simulink model "cooked"  (R2024b)
settings: Solver=VariableStepAuto  StartTime=0.0  StopTime=50  RelTol=1e-3
model workspace (MAT data in the model file):
  w_1 = 5
settings Model: Creator=amlak  LastModifiedBy=amlak
settings DebuggingCC: AlgebraicLoopMsg=none

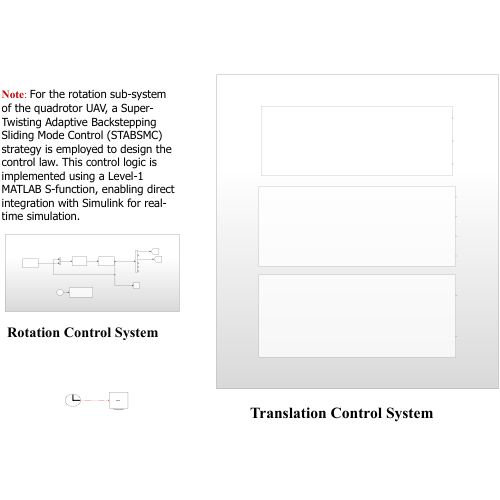
[thumbnail: Simulink's stored preview of the top-level diagram]
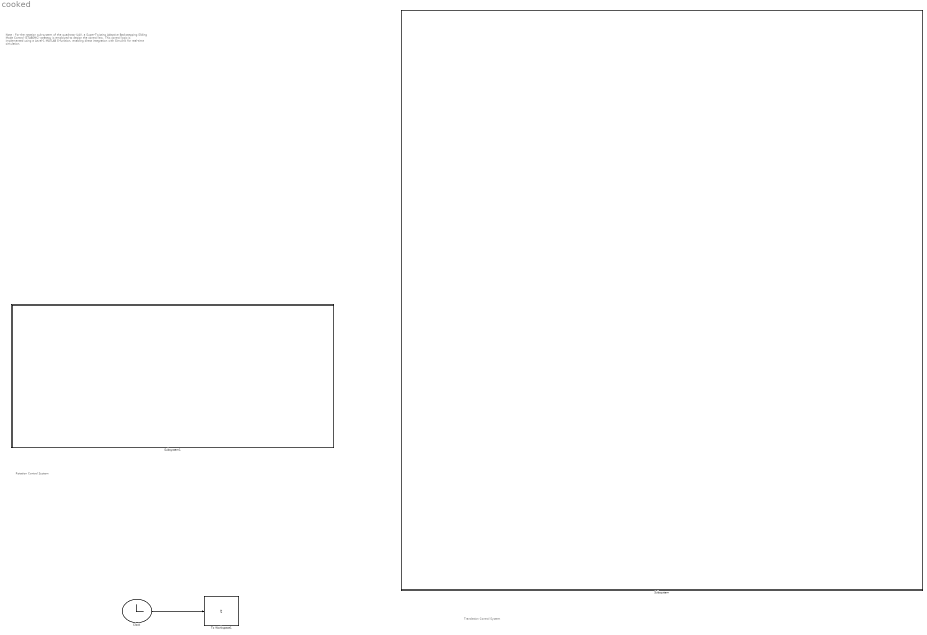
== system cooked ==
  note: Rotation Control System
  note: Note : For the rotation sub-system of the quadrotor UAV, a Super-Twisting Adaptive Backstepping Sliding Mode Control (STABSMC) strategy is employed to design the control law. This control logic is implemented using a Level-1 MATLAB S-function, enabling direct integration with Simulink for real-time simulation.
  note: Translation Control System
  Clock : Clock
      settings: Decimation=50
  Subsystem : Subsystem
  Subsystem1 : Subsystem
  To Workspace1 : ToWorkspace  VariableName=t  SampleTime=-1
      settings: Save2DSignal=2-D array (concatenate along first dimension)
  wires:
  Clock/1 -> To Workspace1/1

== system cooked/Subsystem ==
  Subsystem1 : Subsystem
  Subsystem2 : Subsystem
  Subsystem4 : Subsystem

== system cooked/Subsystem1 ==
  Clock1 : Clock
      settings: Decimation=50
  Demux : Demux  Outputs=6
  Mux1 : Mux  Inputs=2
  S-Function : S-Function  FunctionName=input_qpr  SFunctionDeploymentMode=off  EnableBusSupport=off
  S-Function1 : S-Function  FunctionName=control_qpr  SFunctionDeploymentMode=off  EnableBusSupport=off
  S-Function2 : S-Function  FunctionName=plant_pqr  SFunctionDeploymentMode=off  EnableBusSupport=off
  Scope1 : Scope
  To Workspace : ToWorkspace  VariableName=simout  SaveFormat=Timeseries  SampleTime=-1
  tag scope: x1=global, x3=global
  wires:
  S-Function/1 -> Mux1/2
  Mux1/1 -> S-Function1/1
  Clock1/1 -> To Workspace/1
  S-Function2/1 -> Mux1/1, Scope1/1, Demux/1
  S-Function1/1 -> S-Function2/1
  Demux/3 -> [x3]
  Demux/1 -> [x1]

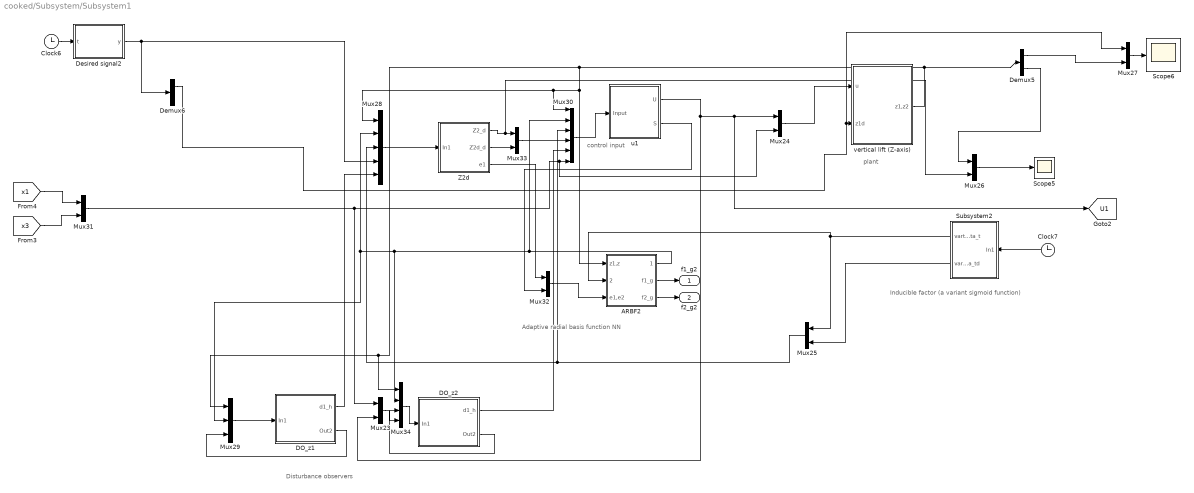
== system cooked/Subsystem/Subsystem1 ==
  note: control input
  note: Inducible factor (a variant sigmoid function)
  note: plant
  note: Disturbance observers
  note: Adaptive radial basis function NN
  ARBF2 : Subsystem
  Clock6 : Clock
      settings: Decimation=50
  Clock7 : Clock
      settings: Decimation=50
  DO_z1 : Subsystem
  DO_z2 : Subsystem
  Demux5 : Demux  Outputs=2
  Demux6 : Demux  Outputs=2
  Desired signal2 : MATLAB Function  TreatAsAtomicUnit=on
  Mux{23..27,31..33} (8 alike) : Mux  Inputs=2
  Mux28 : Mux  Inputs=5
  Mux29 : Mux  Inputs=3
  Mux30 : Mux  Inputs=6
  Mux34 : Mux
  Scope5 : Scope
  Scope6 : Scope
  Subsystem2 : Subsystem
  Z2d : Subsystem
  u1 : Subsystem
  vertical lift (Z-axis) : Subsystem
  f1_g2 : Outport
  f2_g2 : Outport  Port=2
  tag scope: U1=global
  wires:
  u1/1(U) -> Mux23/2, [U1], Mux24/1
  Z2d/3(e1) -> Mux32/1
  vertical lift (Z-axis)/1(z1,z2) -> Mux28/1, Mux30/1, ARBF2/1(z1,z), Mux34/1, Mux29/1, Demux5/1
  Mux26/1 -> Scope5/1
  Mux31/1 -> Mux24/2, Mux30/6, Mux23/1
  ARBF2/2(f1_g) -> f1_g2/1
  Mux24/1 -> vertical lift (Z-axis)/1(u)
  ARBF2/1(lambda) -> Mux30/2, Mux28/2, Mux29/2, Mux34/2
  ARBF2/3(f2_g) -> f2_g2/1
  DO_z2/1(d1_h) -> Mux30/5
  Subsystem2/1(vartheta_t) -> ARBF2/2(vartheta_t), Mux25/1
  Demux5/2 -> Mux26/1
  DO_z1/1(d1_h) -> Mux28/5
  Mux33/1 -> Mux30/4
  Mux32/1 -> ARBF2/3(e1,e2)
  Demux6/1 -> Mux27/1, vertical lift (Z-axis)/2(z1d)
  Mux30/1 -> u1/1(Input)
  Mux28/1 -> Z2d/1(In1)
  Clock7/1 -> Subsystem2/1(In1)
  Z2d/2(Z2d_d) -> Mux33/2
  [x1] -> Mux31/1
  Mux23/1 -> Mux34/4
  DO_z2/2(Out2) -> Mux34/3
  Desired signal2/1(y) -> Demux6/1, Mux28/4
  Mux34/1 -> DO_z2/1(In1)
  Subsystem2/2(vartheta_td) -> Mux25/2
  [x3] -> Mux31/2
  Mux27/1 -> Scope6/1
  Mux29/1 -> DO_z1/1(In1)
  DO_z1/2(Out2) -> Mux29/3
  Z2d/1(Z2_d) -> Mux26/2, Mux33/1
  u1/2(S) -> Mux32/2
  Clock6/1 -> Desired signal2/1(t)
  Demux5/1 -> Mux27/2
  Mux25/1 -> Mux28/3, Mux30/3

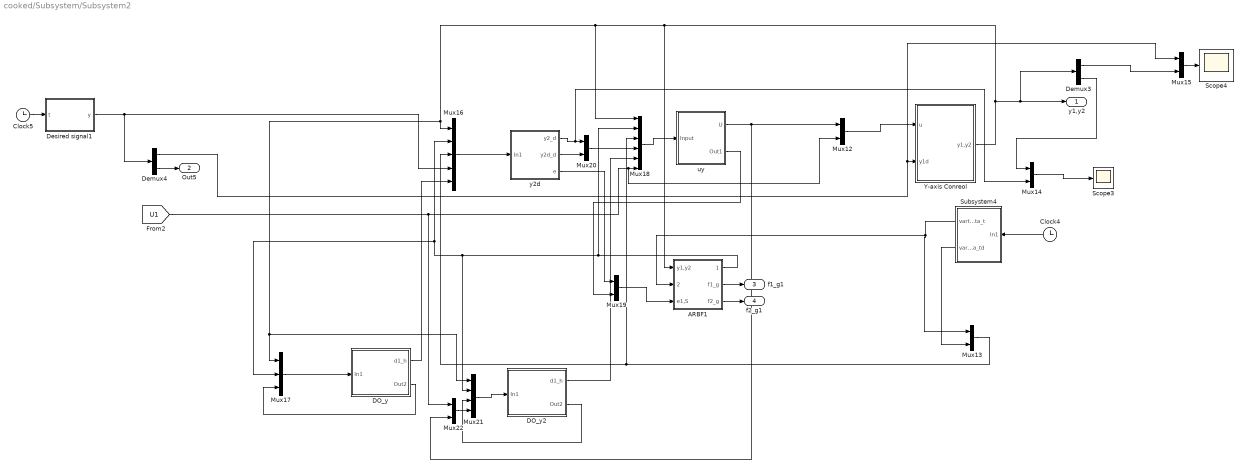
== system cooked/Subsystem/Subsystem2 ==
  ARBF1 : Subsystem
  Clock4 : Clock
      settings: Decimation=50
  Clock5 : Clock
      settings: Decimation=50
  DO_y : Subsystem
  DO_y2 : Subsystem
  Demux3 : Demux  Outputs=2
  Demux4 : Demux  Outputs=2
  Desired signal1 : MATLAB Function  TreatAsAtomicUnit=on
  Mux{12..15,19..20,22} (7 alike) : Mux  Inputs=2
  Mux16 : Mux  Inputs=5
  Mux17 : Mux  Inputs=3
  Mux18 : Mux  Inputs=6
  Mux21 : Mux
  Scope3 : Scope
  Scope4 : Scope
  Subsystem4 : Subsystem
  Y-axis Conreol : Subsystem
  uy : Subsystem
  y2d : Subsystem
  y1,y2 : Outport
  Out5 : Outport  Port=2
  f1_g1 : Outport  Port=3
  f2_g1 : Outport  Port=4
  wires:
  DO_y2/2(Out2) -> Mux21/3
  ARBF1/3(f2_g) -> f2_g1/1
  Mux19/1 -> ARBF1/3(e1,S)
  Clock5/1 -> Desired signal1/1(t)
  Subsystem4/1(vartheta_t) -> Mux13/1, ARBF1/2(vartheta_t)
  Mux16/1 -> y2d/1(In1)
  ARBF1/1(lambda) -> Mux18/2, Mux21/2, Mux17/2, Mux16/2
  Y-axis Conreol/1(y1,y2) -> y1,y2/1, Demux3/1, ARBF1/1(y1,y2), Mux18/1, Mux21/1, Mux17/1, Mux16/1
  Desired signal1/1(y) -> Demux4/1, Mux16/4
  Demux3/2 -> Mux14/1
  Demux4/2 -> Out5/1
  Mux21/1 -> DO_y2/1(In1)
  Mux18/1 -> uy/1(Input)
  [U1] -> Mux12/2, Mux18/6, Mux22/1
  Mux14/1 -> Scope3/1
  Mux17/1 -> DO_y/1(In1)
  y2d/2(y2d_d) -> Mux20/2
  Mux22/1 -> Mux21/4
  Mux13/1 -> Mux16/3, Mux18/3
  y2d/1(y2_d) -> Mux14/2, Mux20/1
  Demux4/1 -> Mux15/1, Y-axis Conreol/2(y1d)
  uy/1(U) -> Mux22/2, Mux12/1
  y2d/3(e) -> Mux19/1
  Clock4/1 -> Subsystem4/1(In1)
  Demux3/1 -> Mux15/2
  DO_y/1(d1_h) -> Mux16/5
  Subsystem4/2(vartheta_td) -> Mux13/2
  DO_y/2(Out2) -> Mux17/3
  Mux20/1 -> Mux18/4
  ARBF1/2(f1_g) -> f1_g1/1
  DO_y2/1(d1_h) -> Mux18/5
  uy/2(Out1) -> Mux19/2
  Mux15/1 -> Scope4/1
  Mux12/1 -> Y-axis Conreol/1(u)

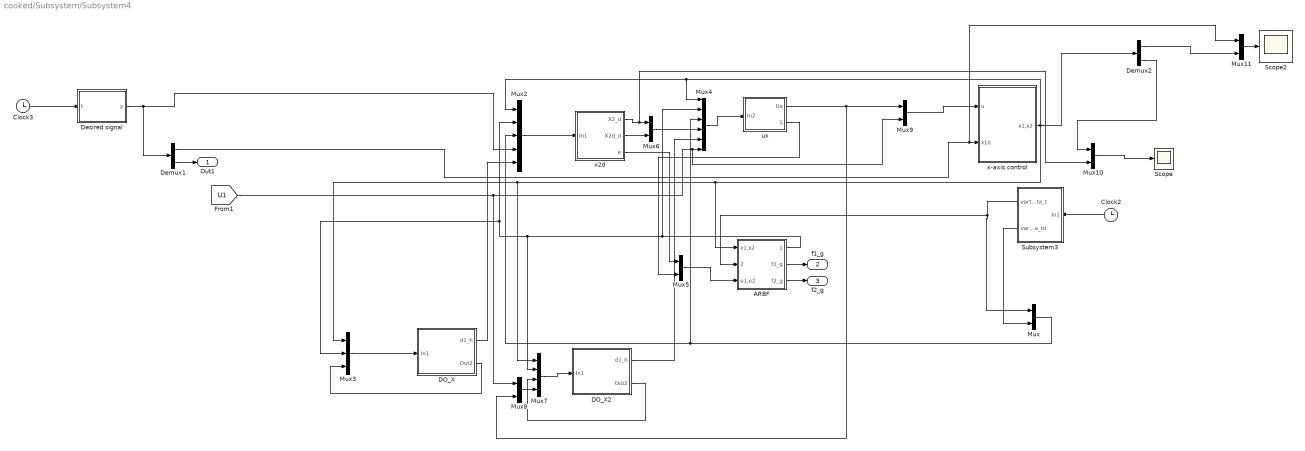
== system cooked/Subsystem/Subsystem4 ==
  ARBF : Subsystem
  Clock2 : Clock
      settings: Decimation=50
  Clock3 : Clock
      settings: Decimation=50
  DO_X : Subsystem
  DO_X2 : Subsystem
  Demux1 : Demux  Outputs=2
  Demux2 : Demux  Outputs=2
  Desired signal : MATLAB Function  TreatAsAtomicUnit=on
  Mux{,5..6,8..11} (7 alike) : Mux  Inputs=2
  Mux2 : Mux  Inputs=5
  Mux3 : Mux  Inputs=3
  Mux4 : Mux  Inputs=6
  Mux7 : Mux
  Scope : Scope
  Scope2 : Scope
  Subsystem3 : Subsystem
  ux : Subsystem
  x-axis control : Subsystem
  x2d : Subsystem
  Out1 : Outport
  f1_g : Outport  Port=2
  f2_g : Outport  Port=3
  wires:
  DO_X/2(Out2) -> Mux3/3
  Mux10/1 -> Scope/1
  ARBF/3(f2_g) -> f2_g/1
  ARBF/1(lambda) -> Mux4/2, Mux7/2, Mux3/2, Mux2/2
  Demux2/2 -> Mux10/1
  Mux3/1 -> DO_X/1(In1)
  Subsystem3/1(vartheta_t) -> Mux/1, ARBF/2(vartheta_t)
  Demux1/1 -> Mux11/1, x-axis control/2(x1d)
  Desired signal/1(y) -> Demux1/1, Mux2/4
  Demux1/2 -> Out1/1
  DO_X2/1(d1_h) -> Mux4/5
  x-axis control/1(x1,x2) -> Mux7/1, Mux3/1, ARBF/1(x1,x2), Demux2/1, Mux2/1, Mux4/1
  DO_X2/2(Out2) -> Mux7/3
  ux/2(S) -> Mux5/2
  [U1] -> Mux9/2, Mux4/6, Mux8/1
  Demux2/1 -> Mux11/2
  Mux5/1 -> ARBF/3(e1,e2)
  Mux9/1 -> x-axis control/1(u)
  Mux2/1 -> x2d/1(In1)
  Subsystem3/2(vartheta_td) -> Mux/2
  Clock3/1 -> Desired signal/1(t)
  DO_X/1(d1_h) -> Mux2/5
  x2d/1(X2_d) -> Mux10/2, Mux6/1
  Mux7/1 -> DO_X2/1(In1)
  x2d/2(X2d_d) -> Mux6/2
  ARBF/2(f1_g) -> f1_g/1
  Mux4/1 -> ux/1(In2)
  Mux6/1 -> Mux4/4
  ux/1(Ux) -> Mux9/1, Mux8/2
  Mux11/1 -> Scope2/1
  Mux8/1 -> Mux7/4
  Mux/1 -> Mux2/3, Mux4/3
  Clock2/1 -> Subsystem3/1(In1)
  x2d/3(e) -> Mux5/1

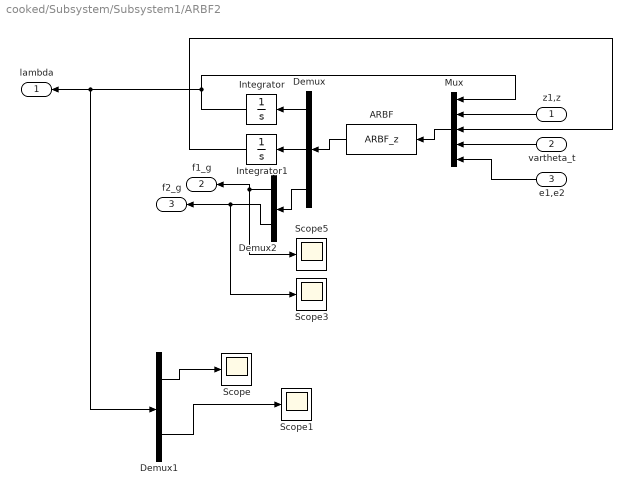
== system cooked/Subsystem/Subsystem1/ARBF2 ==
  z1,z : Inport
  vartheta_t : Inport  Port=2
  e1,e2 : Inport  Port=3
  ARBF : MATLABFcn  MATLABFcn=ARBF_z  OutputDimensions=42
  Demux : Demux  Outputs=[2 38 2]
  Demux1 : Demux  Outputs=2
  Demux2 : Demux  Outputs=2
  Integrator : Integrator
  Integrator1 : Integrator
  Mux : Mux  Inputs=5
  Scope{,1,3,5} (4 alike) : Scope
  lambda : Outport
  f1_g : Outport  Port=2
  f2_g : Outport  Port=3
  wires:
  ARBF/1 -> Demux/1
  Mux/1 -> ARBF/1
  Demux2/1 -> f1_g/1, Scope5/1
  Demux2/2 -> f2_g/1, Scope3/1
  Demux1/1 -> Scope/1
  Demux/1 -> Integrator/1
  Demux/3 -> Demux2/1
  z1,z/1 -> Mux/2
  e1,e2/1 -> Mux/5
  Integrator/1 -> lambda/1, Demux1/1, Mux/1
  Demux/2 -> Integrator1/1
  Demux1/2 -> Scope1/1
  Integrator1/1 -> Mux/3
  vartheta_t/1 -> Mux/4

== system cooked/Subsystem/Subsystem1/DO_z1 ==
  In1 : Inport
  DO1 : MATLABFcn  MATLABFcn=DO_z  OutputDimensions=2
  Demux : Demux  Outputs=2
  Integrator : Integrator
  Scope : Scope
  d1_h : Outport
  Out2 : Outport  Port=2
  wires:
  Demux/2 -> Integrator/1
  DO1/1 -> Demux/1
  In1/1 -> DO1/1
  Integrator/1 -> Out2/1
  Demux/1 -> Scope/1, d1_h/1

== system cooked/Subsystem/Subsystem1/DO_z2 ==
  In1 : Inport
  DO_x2 : MATLABFcn  MATLABFcn=DO_z2  OutputDimensions=2
  Demux : Demux  Outputs=2
  Integrator : Integrator
  d1_h : Outport
  Out2 : Outport  Port=2
  wires:
  Demux/1 -> d1_h/1
  Demux/2 -> Integrator/1
  DO_x2/1 -> Demux/1
  In1/1 -> DO_x2/1
  Integrator/1 -> Out2/1

== system cooked/Subsystem/Subsystem1/Subsystem2 ==
  In1 : Inport
  Demux4 : Demux  Outputs=[1 1]
  Integrator2 : Integrator  InitialCondition=[0 0]
  Mux8 : Mux  Inputs=[1 2]
  filter1 : MATLABFcn  MATLABFcn=filter1
  vartheta : MATLABFcn  MATLABFcn=vartheta_t
  vartheta_t : Outport
  vartheta_td : Outport  Port=2
  wires:
  vartheta/1 -> vartheta_t/1, Mux8/1
  filter1/1 -> Integrator2/1
  Mux8/1 -> filter1/1
  Integrator2/1 -> Demux4/1, Mux8/2
  In1/1 -> vartheta/1
  Demux4/2 -> vartheta_td/1

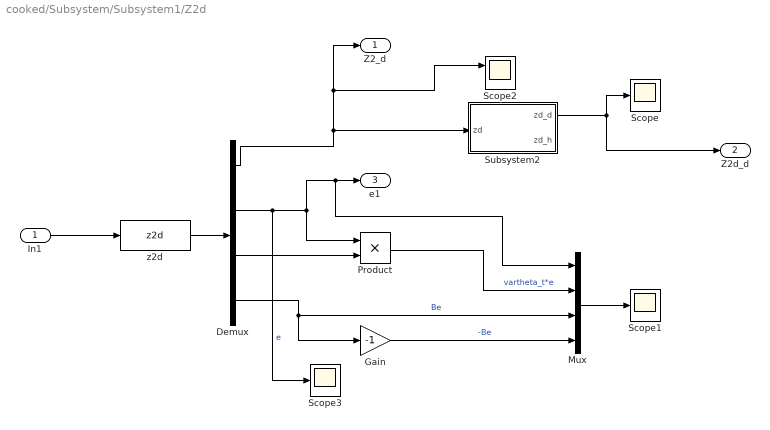
== system cooked/Subsystem/Subsystem1/Z2d ==
  In1 : Inport
  Demux : Demux
  Gain : Gain  Gain=-1
  Mux : Mux
  Product : Product
  Scope : Scope
  Scope1 : Scope
  Scope2 : Scope  NumInputPorts=2
  Scope3 : Scope
  Subsystem2 : Subsystem
  z2d : MATLABFcn  MATLABFcn=z2d  OutputDimensions=4
  Z2_d : Outport
  Z2d_d : Outport  Port=2
  e1 : Outport  Port=3
  wires:
  In1/1 -> z2d/1
  z2d/1 -> Demux/1
  Demux/2 -> Scope3/1, Mux/1, e1/1, Product/1  "e"
  Subsystem2/1(zd_d) -> Z2d_d/1, Scope/1
  Demux/3 -> Product/2
  Demux/4 -> Gain/1, Mux/3  "Be"
  Mux/1 -> Scope1/1
  Product/1 -> Mux/2  "vartheta_t*e"
  Gain/1 -> Mux/4  "-Be"
  Demux/1 -> Scope2/1, Z2_d/1, Subsystem2/1(zd)

== system cooked/Subsystem/Subsystem1/u1 ==
  Input : Inport
  Demux : Demux
  Integrator : Integrator
  Integrator1 : Integrator
  Mux2 : Mux  Inputs=2
  Mux3 : Mux  Inputs=2
  Scope1 : Scope
  Scope3 : Scope
  Scope4 : Scope
  sliding surface : Scope
  u : MATLABFcn  MATLABFcn=u_z  OutputDimensions=4
  U : Outport
  S : Outport  Port=2
  wires:
  u/1 -> Demux/1
  Demux/1 -> Scope1/1, U/1
  Demux/2 -> S/1, sliding surface/1
  Demux/3 -> Integrator1/1
  Demux/4 -> Integrator/1
  Mux2/1 -> Mux3/2
  Mux3/1 -> u/1
  Input/1 -> Mux3/1
  Integrator/1 -> Scope3/1, Mux2/2
  Integrator1/1 -> Scope4/1, Mux2/1

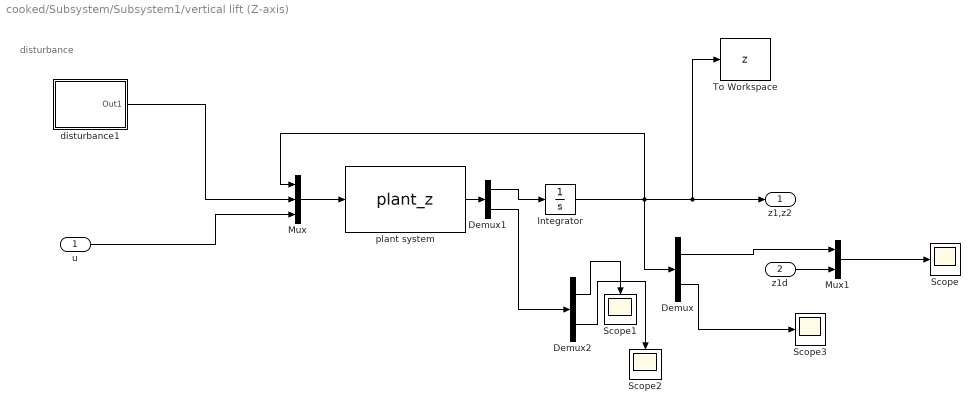
== system cooked/Subsystem/Subsystem1/vertical lift (Z-axis) ==
  note: disturbance
  u : Inport
  z1d : Inport  Port=2
  Demux : Demux  Outputs=2
  Demux1 : Demux  Outputs=[2 2]
  Demux2 : Demux  Outputs=2
  Integrator : Integrator  InitialCondition=[4;1]
  Mux : Mux  Inputs=3
  Mux1 : Mux  Inputs=2
  Scope{,1..3} (4 alike) : Scope
  To Workspace : ToWorkspace  VariableName=z  SampleTime=-1
      settings: Save2DSignal=2-D array (concatenate along first dimension)
  disturbance1 : Subsystem
  plant system : MATLABFcn  MATLABFcn=plant_z  OutputDimensions=4
  z1,z2 : Outport
  wires:
  Mux/1 -> plant system/1
  u/1 -> Mux/3
  disturbance1/1(Out1) -> Mux/2
  Demux/1 -> Mux1/1
  z1d/1 -> Mux1/2
  Mux1/1 -> Scope/1
  Demux/2 -> Scope3/1
  plant system/1 -> Demux1/1
  Demux1/1 -> Integrator/1
  Demux1/2 -> Demux2/1
  Integrator/1 -> Mux/1, Demux/1, To Workspace/1, z1,z2/1
  Demux2/1 -> Scope1/1
  Demux2/2 -> Scope2/1

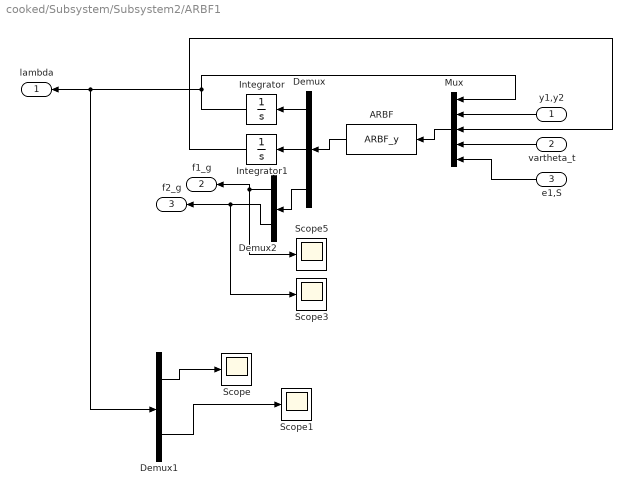
== system cooked/Subsystem/Subsystem2/ARBF1 ==
  y1,y2 : Inport
  vartheta_t : Inport  Port=2
  e1,S : Inport  Port=3
  ARBF : MATLABFcn  MATLABFcn=ARBF_y  OutputDimensions=42
  Demux : Demux  Outputs=[2 38 2]
  Demux1 : Demux  Outputs=2
  Demux2 : Demux  Outputs=2
  Integrator : Integrator
  Integrator1 : Integrator
  Mux : Mux  Inputs=5
  Scope{,1,3,5} (4 alike) : Scope
  lambda : Outport
  f1_g : Outport  Port=2
  f2_g : Outport  Port=3
  wires:
  ARBF/1 -> Demux/1
  Mux/1 -> ARBF/1
  Demux2/1 -> f1_g/1, Scope5/1
  Demux2/2 -> f2_g/1, Scope3/1
  Demux1/1 -> Scope/1
  Demux/1 -> Integrator/1
  Demux/3 -> Demux2/1
  y1,y2/1 -> Mux/2
  e1,S/1 -> Mux/5
  Integrator/1 -> lambda/1, Demux1/1, Mux/1
  Demux/2 -> Integrator1/1
  Demux1/2 -> Scope1/1
  Integrator1/1 -> Mux/3
  vartheta_t/1 -> Mux/4

== system cooked/Subsystem/Subsystem2/DO_y ==
  In1 : Inport
  DO1 : MATLABFcn  MATLABFcn=DO_y  OutputDimensions=2
  Demux : Demux  Outputs=2
  Integrator : Integrator
  d1_h : Outport
  Out2 : Outport  Port=2
  wires:
  Demux/1 -> d1_h/1
  Demux/2 -> Integrator/1
  DO1/1 -> Demux/1
  In1/1 -> DO1/1
  Integrator/1 -> Out2/1

== system cooked/Subsystem/Subsystem2/DO_y2 ==
  In1 : Inport
  DO_x2 : MATLABFcn  MATLABFcn=DO_y2  OutputDimensions=2
  Demux : Demux  Outputs=2
  Integrator : Integrator
  d1_h : Outport
  Out2 : Outport  Port=2
  wires:
  Demux/1 -> d1_h/1
  Demux/2 -> Integrator/1
  DO_x2/1 -> Demux/1
  In1/1 -> DO_x2/1
  Integrator/1 -> Out2/1

== system cooked/Subsystem/Subsystem2/Subsystem4 ==
  In1 : Inport
  Demux4 : Demux  Outputs=[1 1]
  Integrator2 : Integrator  InitialCondition=[0 0]
  Mux8 : Mux  Inputs=[1 2]
  filter1 : MATLABFcn  MATLABFcn=filter1
  vartheta : MATLABFcn  MATLABFcn=vartheta_t
  vartheta_t : Outport
  vartheta_td : Outport  Port=2
  wires:
  vartheta/1 -> vartheta_t/1, Mux8/1
  filter1/1 -> Integrator2/1
  Mux8/1 -> filter1/1
  Integrator2/1 -> Demux4/1, Mux8/2
  In1/1 -> vartheta/1
  Demux4/2 -> vartheta_td/1

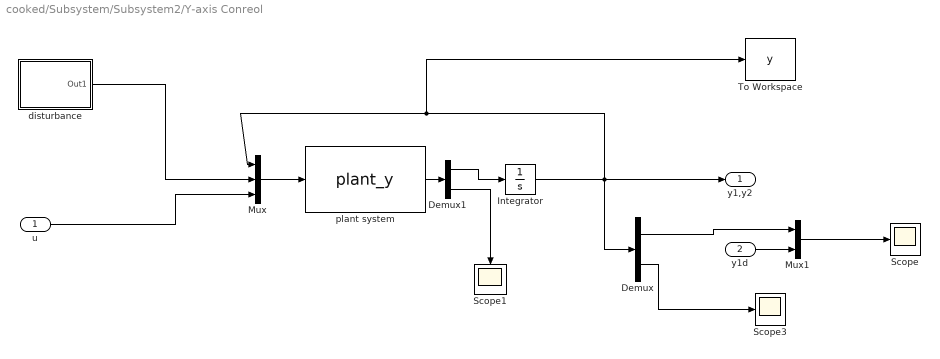
== system cooked/Subsystem/Subsystem2/Y-axis Conreol ==
  u : Inport
  y1d : Inport  Port=2
  Demux : Demux  Outputs=2
  Demux1 : Demux  Outputs=[2 1]
  Integrator : Integrator  InitialCondition=[3;2]
  Mux : Mux  Inputs=3
  Mux1 : Mux  Inputs=2
  Scope : Scope
  Scope1 : Scope
  Scope3 : Scope
  To Workspace : ToWorkspace  VariableName=y  SampleTime=-1
      settings: Save2DSignal=2-D array (concatenate along first dimension)
  disturbance : Subsystem
  plant system : MATLABFcn  MATLABFcn=plant_y  OutputDimensions=3
  y1,y2 : Outport
  wires:
  Mux/1 -> plant system/1
  u/1 -> Mux/3
  disturbance/1(Out1) -> Mux/2
  Demux/1 -> Mux1/1
  y1d/1 -> Mux1/2
  Mux1/1 -> Scope/1
  Demux/2 -> Scope3/1
  plant system/1 -> Demux1/1
  Demux1/1 -> Integrator/1
  Demux1/2 -> Scope1/1
  Integrator/1 -> Mux/1, To Workspace/1, Demux/1, y1,y2/1

== system cooked/Subsystem/Subsystem2/uy ==
  Input : Inport
  Demux : Demux
  Integrator : Integrator
  Integrator1 : Integrator
  Mux2 : Mux  Inputs=2
  Mux3 : Mux  Inputs=2
  Scope : Scope
  Scope1 : Scope
  sliding surface : Scope
  u : MATLABFcn  MATLABFcn=u_y  OutputDimensions=4
  U : Outport
  Out1 : Outport  Port=2
  wires:
  u/1 -> Demux/1
  Demux/1 -> Scope1/1, U/1
  Demux/2 -> Out1/1, sliding surface/1
  Demux/3 -> Integrator1/1
  Demux/4 -> Integrator/1
  Mux2/1 -> Mux3/2
  Mux3/1 -> u/1
  Input/1 -> Mux3/1
  Integrator1/1 -> Mux2/1
  Integrator/1 -> Scope/1, Mux2/2

== system cooked/Subsystem/Subsystem2/y2d ==
  In1 : Inport
  Demux : Demux
  Gain : Gain  Gain=-1
  Mux : Mux
  Product : Product
  Scope : Scope
  Scope1 : Scope
  Scope2 : Scope
  Subsystem2 : Subsystem
  y2d : MATLABFcn  MATLABFcn=y2d  OutputDimensions=4
  y2_d : Outport
  y2d_d : Outport  Port=2
  e : Outport  Port=3
  wires:
  In1/1 -> y2d/1
  y2d/1 -> Demux/1
  Demux/2 -> Mux/1, e/1, Product/1  "e"
  Subsystem2/1(yd_d) -> Scope/1, y2d_d/1
  Demux/3 -> Product/2
  Demux/4 -> Gain/1, Mux/3  "Be"
  Mux/1 -> Scope1/1
  Product/1 -> Mux/2  "vartheta_t*e"
  Gain/1 -> Mux/4  "-Be"
  Demux/1 -> Scope2/1, y2_d/1, Subsystem2/1(y2d)

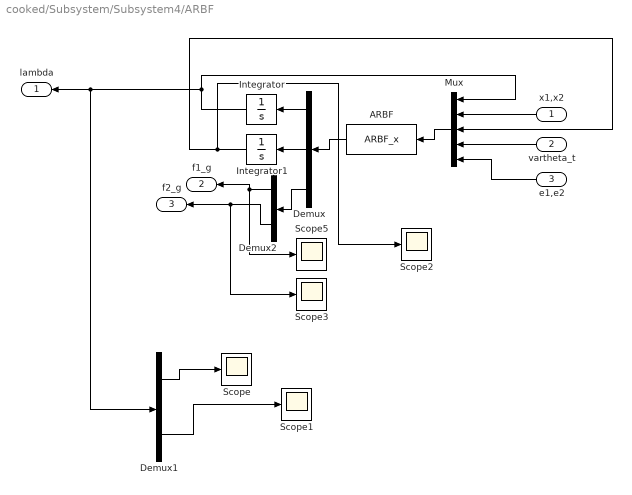
== system cooked/Subsystem/Subsystem4/ARBF ==
  x1,x2 : Inport
  vartheta_t : Inport  Port=2
  e1,e2 : Inport  Port=3
  ARBF : MATLABFcn  MATLABFcn=ARBF_x  OutputDimensions=42
  Demux : Demux  Outputs=[2 38 2]
  Demux1 : Demux  Outputs=2
  Demux2 : Demux  Outputs=2
  Integrator : Integrator
  Integrator1 : Integrator
  Mux : Mux  Inputs=5
  Scope{,1..3,5} (5 alike) : Scope
  lambda : Outport
  f1_g : Outport  Port=2
  f2_g : Outport  Port=3
  wires:
  ARBF/1 -> Demux/1
  Mux/1 -> ARBF/1
  Demux2/1 -> f1_g/1, Scope5/1
  Demux2/2 -> f2_g/1, Scope3/1
  Demux1/1 -> Scope/1
  Demux/1 -> Integrator/1
  Demux/3 -> Demux2/1
  x1,x2/1 -> Mux/2
  e1,e2/1 -> Mux/5
  Integrator/1 -> lambda/1, Demux1/1, Mux/1
  Demux/2 -> Integrator1/1
  Demux1/2 -> Scope1/1
  Integrator1/1 -> Scope2/1, Mux/3
  vartheta_t/1 -> Mux/4

== system cooked/Subsystem/Subsystem4/DO_X ==
  In1 : Inport
  DO1 : MATLABFcn  MATLABFcn=DO_x  OutputDimensions=2
  Demux : Demux  Outputs=2
  Integrator : Integrator
  Scope : Scope
  Scope1 : Scope
  d1_h : Outport
  Out2 : Outport  Port=2
  wires:
  Demux/1 -> Scope/1, d1_h/1
  Demux/2 -> Integrator/1
  DO1/1 -> Demux/1
  In1/1 -> DO1/1
  Integrator/1 -> Scope1/1, Out2/1

== system cooked/Subsystem/Subsystem4/DO_X2 ==
  In1 : Inport
  DO_x2 : MATLABFcn  MATLABFcn=DO_x2  OutputDimensions=2
  Demux : Demux  Outputs=2
  Integrator : Integrator
  d1_h : Outport
  Out2 : Outport  Port=2
  wires:
  Demux/1 -> d1_h/1
  Demux/2 -> Integrator/1
  DO_x2/1 -> Demux/1
  In1/1 -> DO_x2/1
  Integrator/1 -> Out2/1

== system cooked/Subsystem/Subsystem4/Subsystem3 ==
  In1 : Inport
  Demux4 : Demux  Outputs=[1 1]
  Integrator2 : Integrator  InitialCondition=[0 0]
  Mux8 : Mux  Inputs=[1 2]
  filter1 : MATLABFcn  MATLABFcn=filter1
  vartheta : MATLABFcn  MATLABFcn=vartheta_t
  vartheta_t : Outport
  vartheta_td : Outport  Port=2
  wires:
  vartheta/1 -> vartheta_t/1, Mux8/1
  filter1/1 -> Integrator2/1
  Mux8/1 -> filter1/1
  Integrator2/1 -> Demux4/1, Mux8/2
  In1/1 -> vartheta/1
  Demux4/2 -> vartheta_td/1

== system cooked/Subsystem/Subsystem4/ux ==
  In2 : Inport
  Demux2 : Demux
  Integrator : Integrator
  Integrator1 : Integrator
  Mux1 : Mux  Inputs=2
  Mux12 : Mux  Inputs=2
  control Ux : Scope
  sliding surface : Scope
  u : MATLABFcn  MATLABFcn=u_x  OutputDimensions=4
  Ux : Outport
  S : Outport  Port=2
  wires:
  Mux12/1 -> u/1
  u/1 -> Demux2/1
  Integrator1/1 -> Mux1/1
  Demux2/3 -> Integrator1/1
  Mux1/1 -> Mux12/2
  Integrator/1 -> Mux1/2
  Demux2/2 -> S/1, sliding surface/1
  Demux2/4 -> Integrator/1
  Demux2/1 -> control Ux/1, Ux/1
  In2/1 -> Mux12/1

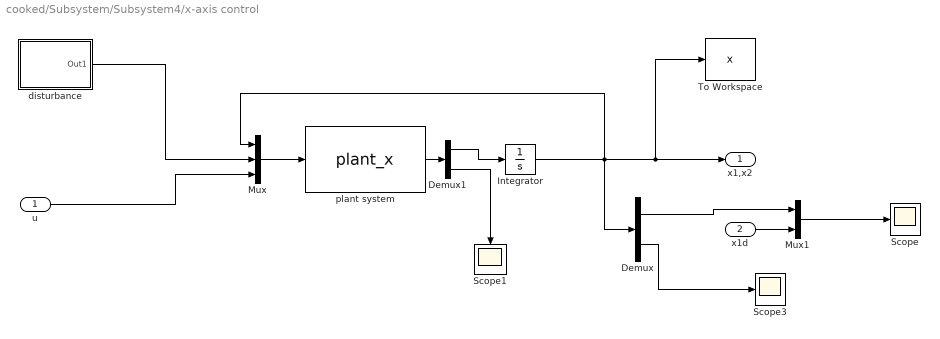
== system cooked/Subsystem/Subsystem4/x-axis control ==
  u : Inport
  x1d : Inport  Port=2
  Demux : Demux  Outputs=2
  Demux1 : Demux  Outputs=[2 1]
  Integrator : Integrator  InitialCondition=[1;2]
  Mux : Mux  Inputs=3
  Mux1 : Mux  Inputs=2
  Scope : Scope
  Scope1 : Scope
  Scope3 : Scope
  To Workspace : ToWorkspace  VariableName=x  SampleTime=-1
      settings: Save2DSignal=2-D array (concatenate along first dimension)
  disturbance : Subsystem
  plant system : MATLABFcn  MATLABFcn=plant_x  OutputDimensions=3
  x1,x2 : Outport
  wires:
  Mux/1 -> plant system/1
  u/1 -> Mux/3
  disturbance/1(Out1) -> Mux/2
  Demux/1 -> Mux1/1
  x1d/1 -> Mux1/2
  Mux1/1 -> Scope/1
  Demux/2 -> Scope3/1
  plant system/1 -> Demux1/1
  Demux1/1 -> Integrator/1
  Demux1/2 -> Scope1/1
  Integrator/1 -> Mux/1, Demux/1, To Workspace/1, x1,x2/1

== system cooked/Subsystem/Subsystem4/x2d ==
  In1 : Inport
  Demux : Demux
  Gain : Gain  Gain=-1
  Mux : Mux
  Product : Product
  Scope{,1..3} (4 alike) : Scope
  Subsystem2 : Subsystem
  x2d : MATLABFcn  MATLABFcn=x2d  OutputDimensions=4
  X2_d : Outport
  X2d_d : Outport  Port=2
  e : Outport  Port=3
  wires:
  In1/1 -> x2d/1
  x2d/1 -> Demux/1
  Demux/2 -> Scope3/1, Mux/1, e/1, Product/1  "e"
  Subsystem2/1(xd_d) -> Scope/1, X2d_d/1
  Demux/3 -> Product/2
  Demux/4 -> Gain/1, Mux/3  "Be"
  Mux/1 -> Scope1/1
  Product/1 -> Mux/2  "vartheta_t*e"
  Gain/1 -> Mux/4  "-Be"
  Demux/1 -> Scope2/1, X2_d/1, Subsystem2/1(xd)

== system cooked/Subsystem/Subsystem1/Z2d/Subsystem2 ==
  zd : Inport
  Demux1 : Demux  Outputs=[1 1]
  Integrator1 : Integrator  InitialCondition=[0 0]
  Mux1 : Mux  Inputs=[1 2]
  filter2 : MATLABFcn  MATLABFcn=filter1  OutputDimensions=2
  zd_d : Outport
  zd_h : Outport  Port=2
  wires:
  filter2/1 -> Integrator1/1
  Mux1/1 -> filter2/1
  Integrator1/1 -> Mux1/2, Demux1/1
  Demux1/2 -> zd_d/1
  Demux1/1 -> zd_h/1
  zd/1 -> Mux1/1

== system cooked/Subsystem/Subsystem1/vertical lift (Z-axis)/disturbance1 ==
  Gain2 : Gain  Gain=5
  Gain3 : Gain
  Gain4 : Gain  Gain=5
  Gain6 : Gain
  Mux1 : Mux  Inputs=3
  Mux3 : Mux  Inputs=2
  Scope : Scope
  d1 : Sin  Amplitude=0  SampleTime=0
  d2 : Sin  Amplitude=0  SampleTime=0
  d3 : Sin  Amplitude=0  SampleTime=0
  d8 : Sin  SampleTime=0
  d9 : Sin  Amplitude=10  SampleTime=0
  Out1 : Outport
  wires:
  Mux3/1 -> Gain2/1
  d8/1 -> Gain6/1
  d9/1 -> Gain3/1
  Gain3/1 -> Mux3/2
  d1/1 -> Mux1/1
  d2/1 -> Mux1/2
  d3/1 -> Gain4/1
  Gain4/1 -> Mux1/3
  Gain2/1 -> Out1/1, Scope/1
  Gain6/1 -> Mux3/1

== system cooked/Subsystem/Subsystem2/Y-axis Conreol/disturbance ==
  Gain2 : Gain  Gain=5
  Gain3 : Gain
  Gain4 : Gain  Gain=5
  Gain6 : Gain
  Mux1 : Mux  Inputs=3
  Mux3 : Mux  Inputs=2
  Scope : Scope
  d1 : Sin  Amplitude=0  SampleTime=0
  d2 : Sin  Amplitude=0  SampleTime=0
  d3 : Sin  Amplitude=0  SampleTime=0
  d8 : Sin  SampleTime=0
  d9 : Sin  Amplitude=10  SampleTime=0
  Out1 : Outport
  wires:
  Mux3/1 -> Gain2/1
  d8/1 -> Gain6/1
  d9/1 -> Gain3/1
  Gain3/1 -> Mux3/2
  d1/1 -> Mux1/1
  d2/1 -> Mux1/2
  d3/1 -> Gain4/1
  Gain4/1 -> Mux1/3
  Gain2/1 -> Out1/1, Scope/1
  Gain6/1 -> Mux3/1

== system cooked/Subsystem/Subsystem2/y2d/Subsystem2 ==
  y2d : Inport
  Demux1 : Demux  Outputs=[1 1]
  Integrator1 : Integrator  InitialCondition=[0 0]
  Mux1 : Mux  Inputs=[1 2]
  filter2 : MATLABFcn  MATLABFcn=filter1
  yd_d : Outport
  yd_h : Outport  Port=2
  wires:
  filter2/1 -> Integrator1/1
  Mux1/1 -> filter2/1
  Integrator1/1 -> Mux1/2, Demux1/1
  Demux1/2 -> yd_d/1
  Demux1/1 -> yd_h/1
  y2d/1 -> Mux1/1

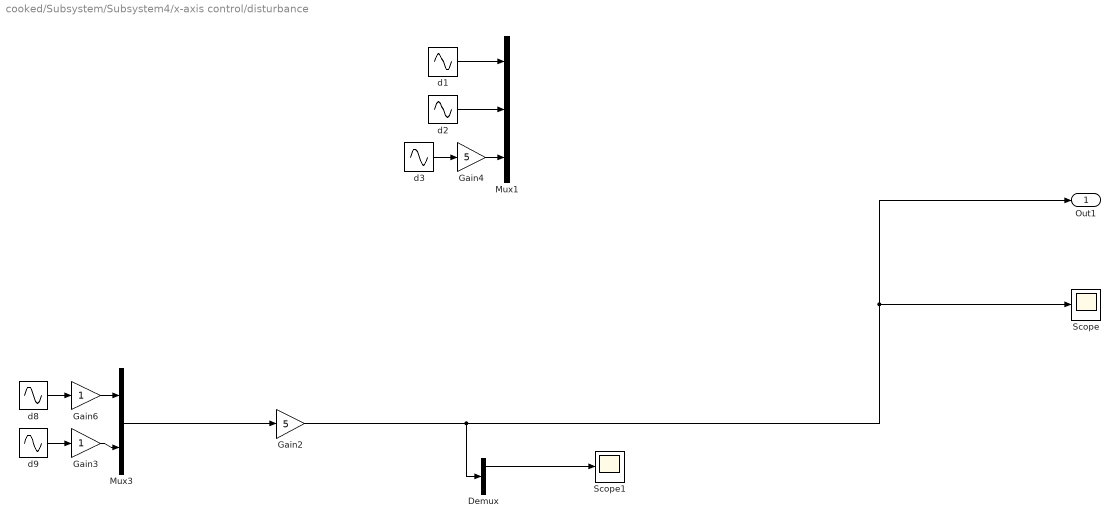
== system cooked/Subsystem/Subsystem4/x-axis control/disturbance ==
  Demux : Demux  Outputs=2
  Gain2 : Gain  Gain=5
  Gain3 : Gain
  Gain4 : Gain  Gain=5
  Gain6 : Gain
  Mux1 : Mux  Inputs=3
  Mux3 : Mux  Inputs=2
  Scope : Scope
  Scope1 : Scope
  d1 : Sin  Amplitude=0  SampleTime=0
  d2 : Sin  Amplitude=0  SampleTime=0
  d3 : Sin  Amplitude=0  SampleTime=0
  d8 : Sin  SampleTime=0
  d9 : Sin  Amplitude=10  SampleTime=0
  Out1 : Outport
  wires:
  Mux3/1 -> Gain2/1
  d8/1 -> Gain6/1
  d9/1 -> Gain3/1
  Gain3/1 -> Mux3/2
  d1/1 -> Mux1/1
  d2/1 -> Mux1/2
  d3/1 -> Gain4/1
  Gain4/1 -> Mux1/3
  Gain2/1 -> Demux/1, Out1/1, Scope/1
  Gain6/1 -> Mux3/1
  Demux/1 -> Scope1/1

== system cooked/Subsystem/Subsystem4/x2d/Subsystem2 ==
  xd : Inport
  Demux1 : Demux  Outputs=[1 1]
  Integrator1 : Integrator  InitialCondition=[0 0]
  Mux1 : Mux  Inputs=[1 2]
  filter2 : MATLABFcn  MATLABFcn=filter1
  xd_d : Outport
  xd_h : Outport  Port=2
  wires:
  filter2/1 -> Integrator1/1
  Mux1/1 -> filter2/1
  Integrator1/1 -> Mux1/2, Demux1/1
  Demux1/2 -> xd_d/1
  Demux1/1 -> xd_h/1
  xd/1 -> Mux1/1

== matlab function cooked/Subsystem/Subsystem2/Desired signal1 ==
  data: t input; y output
function y = fcn(t)

x9d = 5*sin(t);

x9d_d = 5*cos(t);

% x9d_dd = -sin(t)*(3+cos(5*t)) + cos(t)*(5*sin(5*t)) + cos(t)*(-5*sin(5*t)) + sin(t)*(-25*cos(5*t));
y = [x9d, x9d_d]';

== matlab function cooked/Subsystem/Subsystem4/Desired signal ==
  data: t input; y output
function y = fcn(t)

x7d = 5*cos(t);

x7d_d = -5*sin(t);

% x7d_dd = -cos(t)*(3+cos(5*t)) + sin(t)*(5*sin(5*t)) - sin(t)*(-5*sin(5*t)) + cos(t)*(-25*cos(5*t));
y = [x7d, x7d_d]';

== matlab function cooked/Subsystem/Subsystem1/Desired signal2 ==
  data: t input; y output
function y = fcn(t)

x11d = 3*t;

x11d_d = 3;

% x11d_dd = -25*sin(5*t);
y = [x11d, x11d_d]';
